simulink model "OdeSimSpringSimplify"  (R2013a)
settings: Solver=ode45  StartTime=0.0  StopTime=T  MaxStep=1e-4  RelTol=1e-6  AbsTol=1e-6
InitFcn:
  | m=.015;
  | K=1000;
  | L0=.08;
  | f=1;
  | T=1/f;
  | L0_Ode=.1;
  | D_L0_Ode=.02;
  | R=.016;
  | 
  | % Constant Velocity
  | a1=(3/2*pi)/T;
  | 
  | % constant acceleration
  | a2=2*(3/2*pi)/((T^2));
  | 
  | % sin
  | a3=-(3/4*pi);
  | b3=pi/T;
  | c3=pi/2;
  | d3=-a3;
settings Model: Creator=root  LastModifiedBy=root

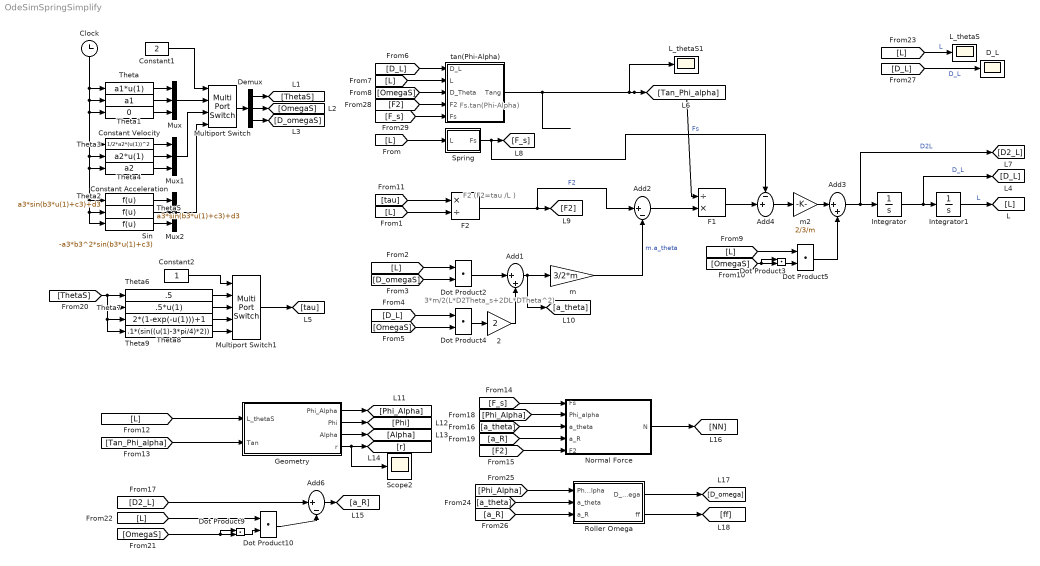
== system OdeSimSpringSimplify ==
  note: 3*m/2(L*D2Theta_s+2DL*DTheta^2)
  note: Fs.tan(Phi-Alpha)
  note: F2 (F2=tau /L )
  2 : Gain  Gain=2
  Add1 : Sum  Inputs=|++
  Add2 : Sum  Inputs=|+-
  Add3 : Sum  Inputs=|++
  Add4 : Sum  Inputs=-+|
  Add6 : Sum  Inputs=|+-
  Clock : Clock
  Constant Acceleration : Fcn  Expr=a2
  Constant Velocity : Fcn  Expr=0
  Constant1 : Constant  Value=2
  Constant2 : Constant
  D_L : Scope
      settings: YMin=-0.0004  YMax=0.0003
  Demux : Demux  Outputs=3
  Dot Product{2..5,9..10} (6 alike) : DotProduct  InputSameDT=on  OutDataTypeStr=Inherit: Inherit via internal rule
  F1 : Product  Inputs=/*
  F2 : Product  Inputs=*/
  Geometry : Subsystem
  Integrator : Integrator  InitialCondition=D_L0_Ode
  Integrator1 : Integrator  InitialCondition=L0_Ode
  L_thetaS : Scope
      settings: YMin=0.055  YMax=0.1  SaveName=ScopeData5
  L_thetaS1 : Scope
      settings: YMin=-0.422  YMax=-0.415
  Multiport Switch : MultiPortSwitch
  Multiport Switch1 : MultiPortSwitch  Inputs=4
  Mux : Mux  Inputs=3
  Mux1 : Mux  Inputs=3
  Mux2 : Mux  Inputs=3
  Normal Force : Subsystem
  Roller Omega : Subsystem
  Scope2 : Scope
      settings: SaveName=ScopeData2
  Sin : Fcn  Expr=-a3*b3^2*sin(b3*u(1)+c3)
  Spring : Subsystem
  Theta : Fcn  Expr=a1*u(1)
  Theta1 : Fcn  Expr=a1
  Theta2 : Fcn  Expr=a3*sin(b3*u(1)+c3)+d3
  Theta3 : Fcn  Expr=1/2*a2*(u(1))^2
  Theta4 : Fcn  Expr=a2*u(1)
  Theta5 : Fcn  Expr=a3*sin(b3*u(1)+c3)+d3
  Theta6 : Fcn  Expr=.5
  Theta7 : Fcn  Expr=.5*u(1)
  Theta8 : Fcn  Expr=2*(1-exp(-u(1)))+1
  Theta9 : Fcn  Expr=.1*(sin((u(1)-3*pi/4)*2))
  m : Gain  Gain=3/2*m
  m2 : Gain  Gain=2/3/m
  tan(Phi-Alpha) : Subsystem
  wires:
  Integrator1/1 -> [L]  "L"
  [L] -> Spring/1(L)
  Spring/1(Fs) -> Add4/1, [F_s]  "Fs"
  tan(Phi-Alpha)/1(Tang) -> L_thetaS1/1, F1/1, [Tan_Phi_alpha]
  [tau] -> F2/1
  [L] -> F2/2
  [L] -> Dot Product2/1
  [D_omegaS] -> Dot Product2/2
  [OmegaS] -> Dot Product4/2
  [D_L] -> Dot Product4/1
  Dot Product4/1 -> 2/1
  Dot Product2/1 -> Add1/1
  2/1 -> Add1/2
  Add1/1 -> m/1, [a_theta]
  Add2/1 -> F1/2
  [L] -> tan(Phi-Alpha)/2(L)
  [D_L] -> tan(Phi-Alpha)/1(D_L)
  Integrator/1 -> [D_L], Integrator1/1  "D_L"
  [OmegaS] -> tan(Phi-Alpha)/3(D_Theta)
  [OmegaS] -> Dot Product3/2, Dot Product3/1
  Dot Product3/1 -> Dot Product5/2
  Add3/1 -> [D2_L], Integrator/1  "D2L"
  [L] -> Dot Product5/1
  [L] -> Geometry/1(L_thetaS)
  [Tan_Phi_alpha] -> Geometry/2(Tan)
  [D2_L] -> Add6/1
  Dot Product10/1 -> Add6/2
  [OmegaS] -> Dot Product9/2, Dot Product9/1
  Dot Product9/1 -> Dot Product10/2
  [L] -> Dot Product10/1
  [F_s] -> Normal Force/1(Fs)
  [a_theta] -> Normal Force/3(a_theta)
  [F2] -> Normal Force/5(F2)
  Normal Force/1(N) -> [NN]
  Geometry/1(Phi_Alpha) -> [Phi_Alpha]
  Geometry/2(Phi) -> [Phi]
  Geometry/3(Alpha) -> [Alpha]
  Geometry/4(r) -> Scope2/1, [r]
  [Phi_Alpha] -> Normal Force/2(Phi_alpha)
  Add6/1 -> [a_R]
  [a_R] -> Normal Force/4(a_R)
  [Phi_Alpha] -> Roller Omega/1(Phi_Alpha)
  [a_theta] -> Roller Omega/2(a_theta)
  [a_R] -> Roller Omega/3(a_R)
  Roller Omega/1(D_omega) -> [D_omega]
  F2/1 -> Add2/1, [F2]  "F2"
  Theta/1 -> Mux/1
  Theta1/1 -> Mux/2
  Constant Velocity/1 -> Mux/3
  Constant1/1 -> Multiport Switch/1
  Mux/1 -> Multiport Switch/2
  Multiport Switch/1 -> Demux/1
  Demux/1 -> [ThetaS]
  Demux/2 -> [OmegaS]
  Demux/3 -> [D_omegaS]
  Theta3/1 -> Mux1/1
  Theta4/1 -> Mux1/2
  Constant Acceleration/1 -> Mux1/3
  Mux1/1 -> Multiport Switch/3
  Clock/1 -> Theta4/1, Sin/1, Theta5/1, Theta2/1, Constant Acceleration/1, Theta3/1, Constant Velocity/1, Theta1/1, Theta/1
  Theta2/1 -> Mux2/1
  Theta5/1 -> Mux2/2
  Sin/1 -> Mux2/3
  Mux2/1 -> Multiport Switch/4
  Multiport Switch1/1 -> [tau]
  Theta6/1 -> Multiport Switch1/2
  Theta7/1 -> Multiport Switch1/3
  Theta8/1 -> Multiport Switch1/4
  Theta9/1 -> Multiport Switch1/5
  Constant2/1 -> Multiport Switch1/1
  [ThetaS] -> Theta9/1, Theta8/1, Theta7/1, Theta6/1
  Roller Omega/2(ff) -> [ff]
  [L] -> L_thetaS/1  "L"
  [D_L] -> D_L/1  "D_L"
  Dot Product5/1 -> Add3/2
  m/1 -> Add2/2  "m.a_theta"
  F1/1 -> Add4/2
  Add4/1 -> m2/1
  m2/1 -> Add3/1
  [F2] -> tan(Phi-Alpha)/4(F2)
  [F_s] -> tan(Phi-Alpha)/5(Fs)

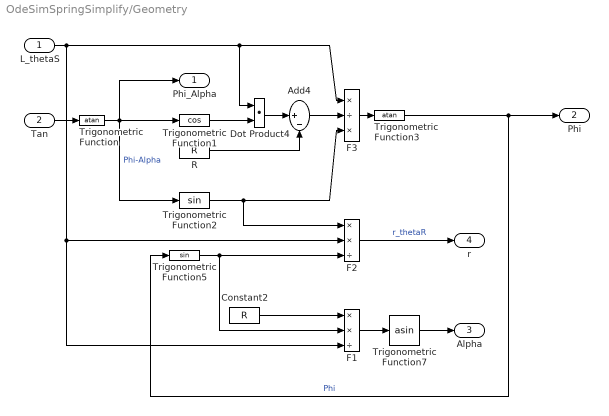
== system OdeSimSpringSimplify/Geometry ==
  L_thetaS : Inport
  Tan : Inport  Port=2
  Add4 : Sum  Inputs=|+-
  Constant2 : Constant  Value=R
  Dot Product4 : DotProduct  InputSameDT=on  OutDataTypeStr=Inherit: Inherit via internal rule
  F1 : Product  Inputs=**/
  F2 : Product  Inputs=**/
  F3 : Product  Inputs=*/*
  R : Constant  Value=R
  Trigonometric Function : Trigonometry  Operator=atan
  Trigonometric Function1 : Trigonometry  Operator=cos
  Trigonometric Function2 : Trigonometry
  Trigonometric Function3 : Trigonometry  Operator=atan
  Trigonometric Function5 : Trigonometry
  Trigonometric Function7 : Trigonometry  Operator=asin
  Phi_Alpha : Outport
  Phi : Outport  Port=2
  Alpha : Outport  Port=3
  r : Outport  Port=4
  wires:
  Tan/1 -> Trigonometric Function/1
  R/1 -> Add4/2
  L_thetaS/1 -> F3/1, Dot Product4/1, F1/3, F2/2
  Trigonometric Function/1 -> Trigonometric Function2/1, Trigonometric Function1/1, Phi_Alpha/1  "Phi-Alpha"
  Dot Product4/1 -> Add4/1
  Trigonometric Function3/1 -> Trigonometric Function5/1, Phi/1  "Phi"
  F3/1 -> Trigonometric Function3/1
  Trigonometric Function1/1 -> Dot Product4/2
  F2/1 -> r/1  "r_thetaR"
  Constant2/1 -> F1/1
  Trigonometric Function5/1 -> F1/2, F2/3
  F1/1 -> Trigonometric Function7/1
  Trigonometric Function7/1 -> Alpha/1
  Add4/1 -> F3/2
  Trigonometric Function2/1 -> F2/1, F3/3

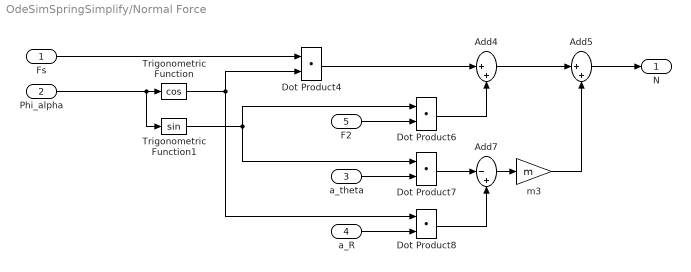
== system OdeSimSpringSimplify/Normal Force ==
  Fs : Inport
  Phi_alpha : Inport  Port=2
  a_theta : Inport  Port=3
  a_R : Inport  Port=4
  F2 : Inport  Port=5
  Add4 : Sum  Inputs=|++
  Add5 : Sum  Inputs=|++
  Add7 : Sum  Inputs=|-+
  Dot Product{4,6..8} (4 alike) : DotProduct  InputSameDT=on  OutDataTypeStr=Inherit: Inherit via internal rule
  Trigonometric Function : Trigonometry  Operator=cos
  Trigonometric Function1 : Trigonometry
  m3 : Gain  Gain=m
  N : Outport
  wires:
  Dot Product6/1 -> Add4/2
  Dot Product8/1 -> Add7/2
  Trigonometric Function/1 -> Dot Product8/1, Dot Product4/2
  m3/1 -> Add5/2
  a_R/1 -> Dot Product8/2
  Add4/1 -> Add5/1
  Dot Product4/1 -> Add4/1
  Dot Product7/1 -> Add7/1
  Add5/1 -> N/1
  Add7/1 -> m3/1
  Phi_alpha/1 -> Trigonometric Function/1, Trigonometric Function1/1
  a_theta/1 -> Dot Product7/2
  Trigonometric Function1/1 -> Dot Product7/1, Dot Product6/1
  F2/1 -> Dot Product6/2
  Fs/1 -> Dot Product4/1

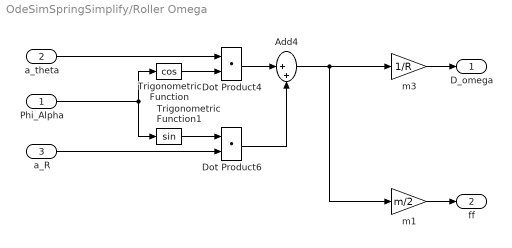
== system OdeSimSpringSimplify/Roller Omega ==
  Phi_Alpha : Inport
  a_theta : Inport  Port=2
  a_R : Inport  Port=3
  Add4 : Sum  Inputs=|++
  Dot Product4 : DotProduct  InputSameDT=on  OutDataTypeStr=Inherit: Inherit via internal rule
  Dot Product6 : DotProduct  InputSameDT=on  OutDataTypeStr=Inherit: Inherit via internal rule
  Trigonometric Function : Trigonometry  Operator=cos
  Trigonometric Function1 : Trigonometry
  m1 : Gain  Gain=m/2
  m3 : Gain  Gain=1/R
  D_omega : Outport
  ff : Outport  Port=2
  wires:
  Dot Product6/1 -> Add4/2
  m3/1 -> D_omega/1
  Add4/1 -> m1/1, m3/1
  Trigonometric Function1/1 -> Dot Product6/1
  Phi_Alpha/1 -> Trigonometric Function/1, Trigonometric Function1/1
  a_R/1 -> Dot Product6/2
  Dot Product4/1 -> Add4/1
  a_theta/1 -> Dot Product4/1
  Trigonometric Function/1 -> Dot Product4/2
  m1/1 -> ff/1

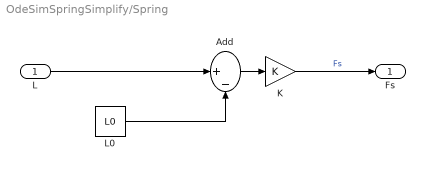
== system OdeSimSpringSimplify/Spring ==
  L : Inport
  Add : Sum  Inputs=|+-
  K : Gain  Gain=K
  L0 : Constant  Value=L0
  Fs : Outport
  wires:
  K/1 -> Fs/1  "Fs"
  Add/1 -> K/1
  L/1 -> Add/1
  L0/1 -> Add/2

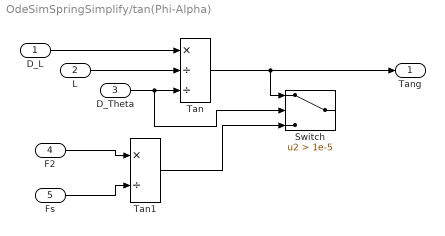
== system OdeSimSpringSimplify/tan(Phi-Alpha) ==
  D_L : Inport
  L : Inport  Port=2
  D_Theta : Inport  Port=3
  F2 : Inport  Port=4
  Fs : Inport  Port=5
  Switch : Switch  Criteria=u2 > Threshold  Threshold=1e-5
  Tan : Product  Inputs=*//
  Tan1 : Product  Inputs=*/
  Tang : Outport
  wires:
  L/1 -> Tan/2
  D_L/1 -> Tan/1
  D_Theta/1 -> Switch/2, Tan/3
  F2/1 -> Tan1/1
  Fs/1 -> Tan1/2
  Tan/1 -> Tang/1, Switch/1
  Tan1/1 -> Switch/3
